simulink model "Parent"  (R2023a)
settings: Solver=FixedStepAuto  StartTime=0.0  StopTime=inf  RelTol=1e-3
undefined symbols (not defined in the file): Data_Display5, Reciever, Size1
libraries: androiduilib x5, androidcommunicationlib x3, androidaudiovideolib x1
settings Model: Creator=Abhishek  LastModifiedBy=Abhishek
settings OptimizationCC: EnhancedBackFolding=on  PassReuseOutputArgsAs=Individual arguments  ZeroExternalMemoryAtStartup=off  ZeroInternalMemoryAtStartup=off  MaxStackSize=64  OptimizeBlockOrder=speed  DifferentSizesBufferReuse=on  OptimizationCustomize=off  EfficientTunableParamExpr=on
settings DebuggingCC: ParameterTunabilityLossMsg=error
settings HardwareCC: ProdBitPerPointer=32  ProdBitPerSizeT=32  ProdBitPerPtrDiffT=32  ProdLargestAtomicInteger=Long  ProdLargestAtomicFloat=Double  ProdWordSize=32  ProdHWDeviceType=ARM Compatible->ARM Cortex  UseEmbeddedCoderFeatures=off  UseSimulinkCoderFeatures=off
settings SFSimCC: MATLABDynamicMemAlloc=off
settings RTWCC: Description=Embedded Coder  SystemTargetFile=ert.tlc  HardwareBoard=Android Device  TLCOptions="-aInlineSetEventsForThisBaseRateFcn=TLC_FALSE -aSuppressMultiTaskScheduler=TLC_FALSE  -aRateBasedStepFcn=0"  TemplateMakefile=ert_default_tmf  RTWVerbose=off  Toolchain=Android SDK/NDK Tools
settings CodeAppCC: ForceParamTrailComments=on  IgnoreCustomStorageClasses=off  OperatorAnnotations=on  SimulinkDataObjDesc=on  SFDataObjDesc=on  InsertBlockDesc=on
settings ERTTargetCC: SupportNonInlinedSFcns=on

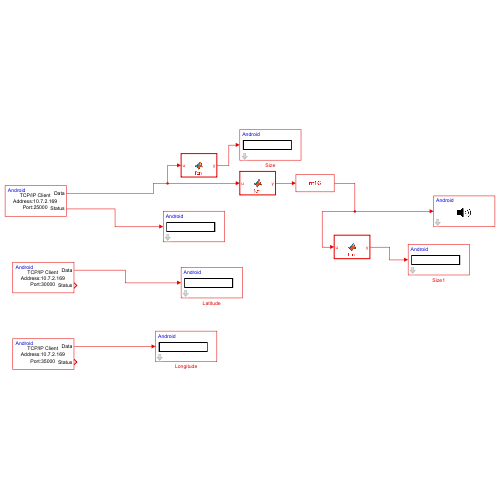
[thumbnail: Simulink's stored preview of the top-level diagram]
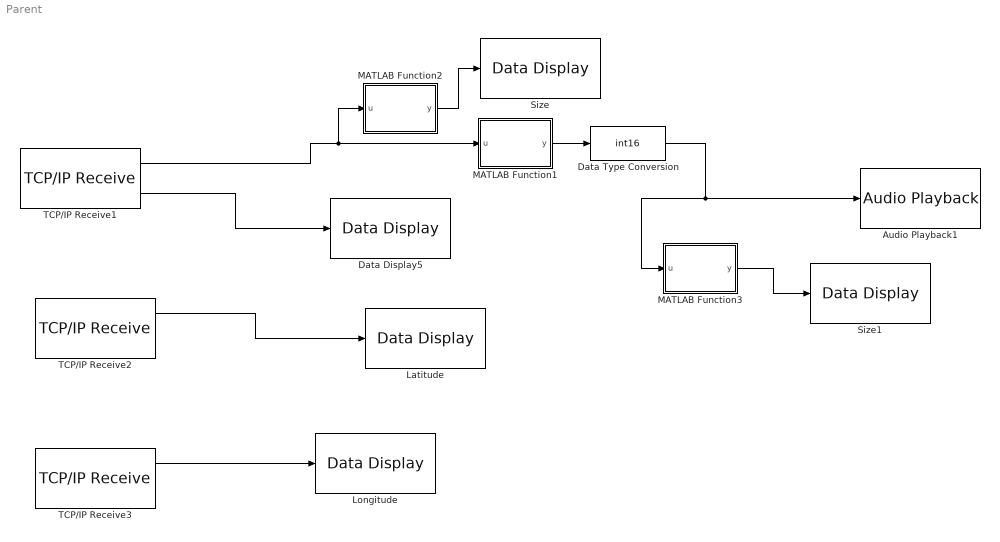
== system Parent ==
  Audio Playback1 : androidaudiovideolib/Audio Playback  SampleFreq=24000  AudioSamplingFreq=24000  SampleTime=0.1  DeviceStr=0  QueueDuration=0  BlockPlatform=Android
  Data Display5 : androiduilib/Data Display  DataDisplayId=Reciever/Data_Display5  Format=Float  Precision=6  SimulateUsing=Code generation  blockPlatform=Android
  Data Type Conversion : DataTypeConversion  OutDataTypeStr=int16  SaturateOnIntegerOverflow=off  RndMeth=Floor
  Latitude : androiduilib/Data Display  DataDisplayId=Reciever/Latitude  Format=Float  Precision=6  SimulateUsing=Code generation  blockPlatform=Android
  Longitude : androiduilib/Data Display  DataDisplayId=Reciever/Longitude  Format=Float  Precision=6  SimulateUsing=Code generation  blockPlatform=Android
  MATLAB Function1 : MATLAB Function  TreatAsAtomicUnit=on
  MATLAB Function2 : MATLAB Function  TreatAsAtomicUnit=on
  MATLAB Function3 : MATLAB Function  TreatAsAtomicUnit=on
  Size : androiduilib/Data Display  DataDisplayId=Reciever/Size  Format=Float  Precision=6  SimulateUsing=Code generation  blockPlatform=Android
  Size1 : androiduilib/Data Display  DataDisplayId=Reciever/Size1  Format=Float  Precision=6  SimulateUsing=Code generation  blockPlatform=Android
  TCP/IP Receive1 : androidcommunicationlib/TCP//IP Receive  TCPReceiveId=Reciever/TCP//IP_Receive1  Mode_=Client  LocalServerPort_=25000  RemoteAddr_=10.7.2.169  RemoteServerPort_=25000  DataType_=double  DataSize_=300  SampleTime_=0.0125  ClientPortBindingSelection_=off  ClientPortToBind_=35000  BlockingMode_=off  BlockTimeout_=0.1
  TCP/IP Receive2 : androidcommunicationlib/TCP//IP Receive  TCPReceiveId=Reciever/TCP//IP_Receive2  Mode_=Client  LocalServerPort_=25000  RemoteAddr_=10.7.2.169  RemoteServerPort_=30000  DataType_=double  DataSize_=1  SampleTime_=0.0125  ClientPortBindingSelection_=off  ClientPortToBind_=35000  BlockingMode_=off  BlockTimeout_=0.1
  TCP/IP Receive3 : androidcommunicationlib/TCP//IP Receive  TCPReceiveId=Reciever/TCP//IP_Receive3  Mode_=Client  LocalServerPort_=25000  RemoteAddr_=10.7.2.169  RemoteServerPort_=35000  DataType_=double  DataSize_=1  SampleTime_=0.0125  ClientPortBindingSelection_=off  ClientPortToBind_=35000  BlockingMode_=off  BlockTimeout_=0.1
  wires:
  TCP/IP Receive3/1 -> Longitude/1
  TCP/IP Receive2/1 -> Latitude/1
  TCP/IP Receive1/2 -> Data Display5/1
  TCP/IP Receive1/1 -> MATLAB Function2/1(u), MATLAB Function1/1(u)
  MATLAB Function1/1(y) -> Data Type Conversion/1
  Data Type Conversion/1 -> Audio Playback1/1, MATLAB Function3/1(u)
  MATLAB Function2/1(y) -> Size/1
  MATLAB Function3/1(y) -> Size1/1

== matlab function Parent/MATLAB Function2 ==
  data: u input; y output
function y = fcn(u)

y = size(u);

== matlab function Parent/MATLAB Function3 ==
  data: u input; y output
function y = fcn(u)

y = size(u);

== matlab function Parent/MATLAB Function1 ==
  data: u input; y output
function y = fcn(u)

y = [u,u];
